simulink model "SEL_test"  (R2026a)
settings: Solver=ode8  StopTime=1  FixedStep=8e-9
PreLoadFcn:
  | setup_llrf
model workspace (MAT data in the model file):
  adc_sample_time = 8e-09
  alpha_ema = 0.00390625
  mag_Ki = 2000
  mag_Kp = 0.5
  max_dac_out = 1
  min_dac_out = 0
values from neighbouring files (symbols this model uses):
  f_IF = 10e6    (= 10000000)    [setup_llrf.m]
  f_sample = 125e6    (= 125000000)    [setup_llrf.m]
  lut_rSqrt = fi(lut_combined_float, 0, WL, FL, 'RoundingMethod', 'Nearest')    [LUT_gen.m]    (also in setup_llrf.m = LUT_gen)
  omega_0 = 2 * pi * f_IF    (= 62831853.0718)    [setup_llrf.m]
  omega_half = (f_0_rf / (2 * Q_L)) * 2 * pi    (= 8168.14089933)    [setup_llrf.m]
  params = extractHDLParams(filt)    [setup_llrf.m]
  t_sample = 1/f_sample    (= 8e-09)    [setup_llrf.m]
libraries: simulink x3, hdlsllib x2, dsphdlfiltering2 x2, dsphdlsigops2 x1
settings Model: DataTypeOverride=Off  FPTShortcutValueString='{{},{''BaselineRun'',1,1,1,''BaselineRun'','''',{},''M'',''D'',''''},{''BaselineRun_2'',1,1,1,''BaselineRun_2'','''',{},''M'',''D'',''''},{''EmbeddedRun'',1,1,1,''EmbeddedRun'','''',{},''M'','''',''''},{''EmbeddedRun_2'',1,1,1,''EmbeddedRun_2'','''',{},''M'','''',''''}}'  SnapshotInterval=1  Creator=Joshd  LastModifiedBy=Joshd
settings DataIOCC: InspectSignalLogs=on
settings OptimizationCC: ConditionallyExecuteInputs=off  InheritOutputTypeSmallerThanSingle=on
settings DebuggingCC: SignalRangeChecking=warning  ArtificialAlgebraicLoopMsg=error  SingleTaskRateTransMsg=error  UniqueDataStoreMsg=error  StrictBusMsg=ErrorOnBusTreatedAsVector
settings HardwareCC: ProdHWDeviceType=ASIC/FPGA->ASIC/FPGA  ProdEqTarget=off
settings ConfigComp: CovScope=ReferencedModels

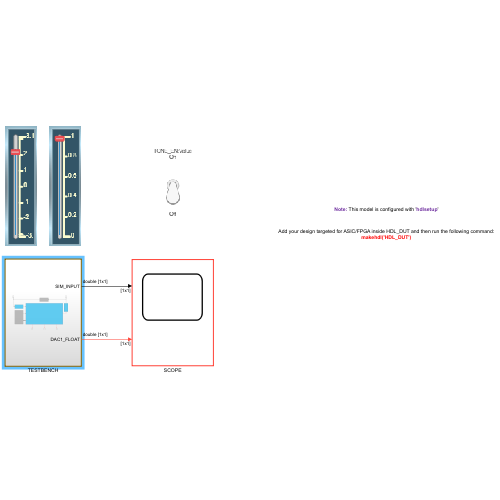
[thumbnail: Simulink's stored preview of the top-level diagram]
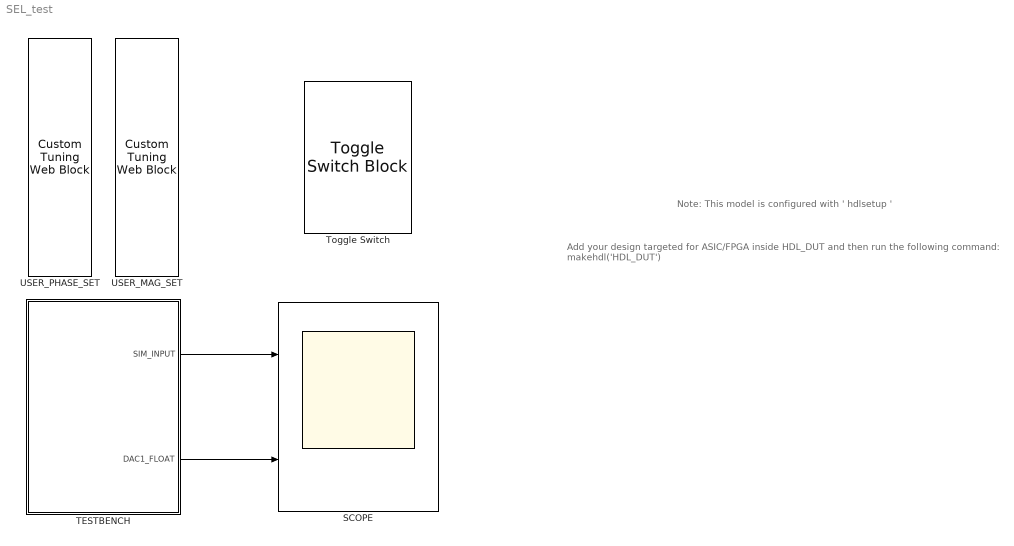
== system SEL_test ==
  note: Add your design targeted for ASIC/FPGA inside HDL_DUT and then run the following command:
      | makehdl('HDL_DUT')
  note: Note: This model is configured with ' hdlsetup '
  SCOPE : Scope  NumInputPorts=2
      settings: TimeSpan=1e-6  ActiveDisplayYMinimum=-2.1650361300192067  ActiveDisplayYMaximum=1.9862346787804239
  TESTBENCH : Subsystem
  Toggle Switch : ToggleSwitchBlock
  USER_MAG_SET : CustomTuningWebBlock  LabelPosition=Hide  ShowInitialText=on  Configuration="{\"components\":[{\"name\":\"LinearScaleComponent\",\"settings\":{\"bounds\":{\"max\":1,\"min\":0,\"tickInterval\":\"auto\"},\"internalTickHeightScaleFactor\":0.5,\"labelColor\":[255,255,200],\"labelFont\":{\"font\":\"Arial\",\"fontSize\":12},\"labelOffset\":0.05,\"labelTransparency\":1,\"needleImage\":{\"size\":[596,842],\"src\":\"data:image\\/svg+xml;base64,PD94bWwgdmVyc2lvbj0iMS4wIiBlbmNvZGluZz0idXRmLTgiPz4NCjwhLS0gR2VuZXJhdG9yOiBBZG9iZSBJbGx1c3RyYXRvciAyNS4wLjAsIFNWRyBFeHBvcnQgUGx1Zy1JbiAuIFNWRyBWZXJzaW9uOiA2LjAwIEJ1aWxkIDApICAtLT4NCjxzdmcgdmVyc2lvbj0iMS4xIg0KCSBpZD0ic3ZnOCIgeG1sbnM6Y2M9Imh0dHA6Ly9jcmVhdGl2ZWNvbW1vbnMub3JnL25zIyIgeG1sbnM6ZGM9Imh0dHA6Ly9wdXJsLm9yZy9kYy9lbGVtZW50cy8xLjEvIiB4bWxuczppbmtzY2FwZT0iaHR0cDovL3d3dy5pbmtzY2FwZS5vcmcvbmFtZXNw ...(+2420 chars)\",\"srcOrientation\":\"horizontal\"},\"needleOffset\":[0.0642123287671233,-0.8044596912521441],\"needleSize\":{\"height\":0.07668067226890757,\"width\":0.4337797619047619},\"position\":[0.03623949579831933,0.2829861111111111,0.6088789682539683,0.9196428571428571],\"referencePoint\":\"auto\",\"scaleColors\":[],\"scaleColorsSize\":0.2,\"scaleDirection\":\"BT\",\"showLabels\":1,\"showMinorTicks\":0,\"showSpanLine\":1,\"showTicks\":1,\"tickColor\":[252,252,197],\"tickTransparency\":1,\"valueBarColor\":[0,114,189],\"valueBarOffset\":-0.27,\"valueBarSize\":0.1,\"valueBarTransparency\":1}},{\"name\":\"BackgroundImageComponent\",\"settings\":{\"image\":{\"size\":[380,101],\"src\":\"data:image\\/svg+xml;base64,PHN2ZyB4bWxucz0iaHR0cDovL3d3dy53My5vcmcvMjAwMC9zdmciIHhtbG5zOnhsaW5rPSJodHRwOi8vd3d3LnczLm9yZy8xOTk5L3hsaW5rIiB2aWV3Qm94PSIwIDAgMzgwIDEwMSI+PGRlZnM+PHN0eWxlPi5jbHMtMXtmaWxsOiMwMDJiNDI7fS5jbHMtMntmaWxsOiM0MjcwODI7fS5jbHMtM3tmaWxsOnVybCgjcmFkaWFsLWdyYWRpZW50KTt9LmNscy00e2ZpbGw6I2M4YzhjODtzdHJva2U6IzAwMDt9PC9zdHlsZT48cmFkaWFsR3JhZGllbnQgaWQ9InJhZGlhbC1ncmFkaWVudCIgY3g9IjE5MCIgY3k9IjUwLjUiIHI9IjI2OS4yMSIgZ3JhZGllbnRVbml0cz0idXNlclNwYWNlT25Vc2UiPjxzdG9wIG9mZnNldD0iMC4wMSIgc3RvcC1jb2xvcj0iIzNlNGY1OCIvPjxzdG9wIG9mZnNldD0iMC4wNiIgc3RvcC1jb2xvcj0iIzQ0NTc2MSIvPjxzdG9wIG9mZnNldD0iMC4xNSIgc3RvcC1jb2xvcj0iIzU1NmE3NiIvPjxzdG9wIG9mZnNldD0iMC4yNSIgc3RvcC1jb2xvcj0iIzZkODg5NSIvPjxzdG9wIG9mZnNldD0iMC4zOCIgc3RvcC1jb2xvcj0iIzhmYjJjMyIvPjxzdG9wIG9mZnNldD0iMC41MiIgc3RvcC1jb2xvcj0iI2I2ZTRmYSIvPjxzdG9wIG9mZnNldD0iMSIgc3RvcC1jb2xvcj0iIzE1NDY1NyIvPjwvcmFkaWFsR3JhZGllbnQ+PC9kZWZzPjxnIGlkPSJmcmFtZSI+PGcgaWQ9IkxheWVyXzIiIGRhdGEtbmFtZT0iTGF5ZXIgMiI+PGcgaWQ9IkxheWVyXzEtMiIgZGF0YS1uYW1lPSJMYXllciAxLTIiPjxyZWN0IGlkPSJyZWN0MTAzNiIgY2xhc3M9ImNscy0xIiB4PSIxMSIgeT0iMTEiIHdpZHRoPSIzNTgiIGhlaWdodD0iNzkiLz48cGF0aCBpZD0icGF0aDEwMzgiIGNsYXNzPSJjbHMtMiIgZD0iTTgsOFY5M0gzNzJWOFpNMzY5LDkwSDExVjExSDM2OVoiLz48cGF0aCBpZD0icGF0aDEwNDAiIGNsYXNzPSJjbHMtMyIgZD0iTTAsMFYxMDFIMzgwVjBaTTM3Miw5M0g4VjhIMzcyWiIvPjwvZz48L2c+PC9nPjxnIGlkPSJ0cmFjayI+PHBhdGggaWQ9InJlY3QxNjExIiBjbGFzcz0iY2xzLTQiIGQ9Ik0zMy4zNywyNi41OUgzNDYuNjNjNCwwLDcuMjUsMi42LDcuMjUsNS44MWgwYzAsMy4yMS0zLjI1LDUuODItNy4yNSw1LjgySDMzLjM3Yy00LDAtNy4yNS0yLjYxLTcuMjUtNS44MmgwQzI2LjEyLDI5LjE5LDI5LjM3LDI2LjU5LDMzLjM3LDI2LjU5WiIvPjwvZz48L3N2Zz4=\",\"srcOrientation\":\"horizontal\"},\"position\":[0,0,1,1],\"scaleMode\":\"0\"}},{\"name\":\"ForegroundImageComponent\",\"settings\":{\"image\":{\"size\":[0,0],\"src\":\"default\",\"srcOrientation\":[]},\"isForeground\":1,\"position\":[0,0,1,1],\"scaleMode\":\"0\"}}],\"derived\":{\"blockParameters\":{\"ForegroundColor\":[0.9882352941176471,0.9882352941176471,0.7725490196078432],\"Limits\":{\"Max\":1,\"Min\":0,\"Ticks\":\"auto\"},\"ScaleColors\":[],\"ScaleDirection\":\"Clockwise\",\"ScaleMax\":1,\"ScaleMin\":0,\"TickInterval\":\"auto\",\"fixedAspectRatio\":\"on\"}},\"settings\":{\"BindingType\":\"param\",\"aspectRatio\":3.7777777777777777,\"backgroundColor\":[0,0,0,\"1\"],\"backgroundOffset\":0,\"backgroundOpacity\":1,\"fixedAspectRatio\":\"on\",\"foregroundColor\":[252,252,196],\"orientation\":\"vertical\",\"showBackgroundColor\":false,\"value\":0,\"version\":\"R2023a\"},\"type\":\"LinearGauge\"}"
  USER_PHASE_SET : CustomTuningWebBlock  LabelPosition=Hide  ShowInitialText=on  Configuration="{\"components\":[{\"name\":\"LinearScaleComponent\",\"settings\":{\"bounds\":{\"max\":3.14159,\"min\":-3.14159,\"tickInterval\":\"auto\"},\"internalTickHeightScaleFactor\":0.5,\"labelColor\":[255,255,200],\"labelFont\":{\"font\":\"Arial\",\"fontSize\":12},\"labelOffset\":0.05,\"labelTransparency\":1,\"needleImage\":{\"size\":[596,842],\"src\":\"data:image\\/svg+xml;base64,PD94bWwgdmVyc2lvbj0iMS4wIiBlbmNvZGluZz0idXRmLTgiPz4NCjwhLS0gR2VuZXJhdG9yOiBBZG9iZSBJbGx1c3RyYXRvciAyNS4wLjAsIFNWRyBFeHBvcnQgUGx1Zy1JbiAuIFNWRyBWZXJzaW9uOiA2LjAwIEJ1aWxkIDApICAtLT4NCjxzdmcgdmVyc2lvbj0iMS4xIg0KCSBpZD0ic3ZnOCIgeG1sbnM6Y2M9Imh0dHA6Ly9jcmVhdGl2ZWNvbW1vbnMub3JnL25zIyIgeG1sbnM6ZGM9Imh0dHA6Ly9wdXJsLm9yZy9kYy9lbGVtZW50cy8xLjEvIiB4bWxuczppbmtzY2FwZT0iaHR0cDovL3d3dy5pbmtzY2FwZS5vcmcvbmFtZXNw ...(+2420 chars)\",\"srcOrientation\":\"horizontal\"},\"needleOffset\":[0.0642123287671233,-0.8044596912521441],\"needleSize\":{\"height\":0.07668067226890757,\"width\":0.4337797619047619},\"position\":[0.03623949579831933,0.2829861111111111,0.6088789682539683,0.9196428571428571],\"referencePoint\":\"auto\",\"scaleColors\":[],\"scaleColorsSize\":0.2,\"scaleDirection\":\"BT\",\"showLabels\":1,\"showMinorTicks\":0,\"showSpanLine\":1,\"showTicks\":1,\"tickColor\":[252,252,197],\"tickTransparency\":1,\"valueBarColor\":[0,114,189],\"valueBarOffset\":-0.27,\"valueBarSize\":0.1,\"valueBarTransparency\":1}},{\"name\":\"BackgroundImageComponent\",\"settings\":{\"image\":{\"size\":[380,101],\"src\":\"data:image\\/svg+xml;base64,PHN2ZyB4bWxucz0iaHR0cDovL3d3dy53My5vcmcvMjAwMC9zdmciIHhtbG5zOnhsaW5rPSJodHRwOi8vd3d3LnczLm9yZy8xOTk5L3hsaW5rIiB2aWV3Qm94PSIwIDAgMzgwIDEwMSI+PGRlZnM+PHN0eWxlPi5jbHMtMXtmaWxsOiMwMDJiNDI7fS5jbHMtMntmaWxsOiM0MjcwODI7fS5jbHMtM3tmaWxsOnVybCgjcmFkaWFsLWdyYWRpZW50KTt9LmNscy00e2ZpbGw6I2M4YzhjODtzdHJva2U6IzAwMDt9PC9zdHlsZT48cmFkaWFsR3JhZGllbnQgaWQ9InJhZGlhbC1ncmFkaWVudCIgY3g9IjE5MCIgY3k9IjUwLjUiIHI9IjI2OS4yMSIgZ3JhZGllbnRVbml0cz0idXNlclNwYWNlT25Vc2UiPjxzdG9wIG9mZnNldD0iMC4wMSIgc3RvcC1jb2xvcj0iIzNlNGY1OCIvPjxzdG9wIG9mZnNldD0iMC4wNiIgc3RvcC1jb2xvcj0iIzQ0NTc2MSIvPjxzdG9wIG9mZnNldD0iMC4xNSIgc3RvcC1jb2xvcj0iIzU1NmE3NiIvPjxzdG9wIG9mZnNldD0iMC4yNSIgc3RvcC1jb2xvcj0iIzZkODg5NSIvPjxzdG9wIG9mZnNldD0iMC4zOCIgc3RvcC1jb2xvcj0iIzhmYjJjMyIvPjxzdG9wIG9mZnNldD0iMC41MiIgc3RvcC1jb2xvcj0iI2I2ZTRmYSIvPjxzdG9wIG9mZnNldD0iMSIgc3RvcC1jb2xvcj0iIzE1NDY1NyIvPjwvcmFkaWFsR3JhZGllbnQ+PC9kZWZzPjxnIGlkPSJmcmFtZSI+PGcgaWQ9IkxheWVyXzIiIGRhdGEtbmFtZT0iTGF5ZXIgMiI+PGcgaWQ9IkxheWVyXzEtMiIgZGF0YS1uYW1lPSJMYXllciAxLTIiPjxyZWN0IGlkPSJyZWN0MTAzNiIgY2xhc3M9ImNscy0xIiB4PSIxMSIgeT0iMTEiIHdpZHRoPSIzNTgiIGhlaWdodD0iNzkiLz48cGF0aCBpZD0icGF0aDEwMzgiIGNsYXNzPSJjbHMtMiIgZD0iTTgsOFY5M0gzNzJWOFpNMzY5LDkwSDExVjExSDM2OVoiLz48cGF0aCBpZD0icGF0aDEwNDAiIGNsYXNzPSJjbHMtMyIgZD0iTTAsMFYxMDFIMzgwVjBaTTM3Miw5M0g4VjhIMzcyWiIvPjwvZz48L2c+PC9nPjxnIGlkPSJ0cmFjayI+PHBhdGggaWQ9InJlY3QxNjExIiBjbGFzcz0iY2xzLTQiIGQ9Ik0zMy4zNywyNi41OUgzNDYuNjNjNCwwLDcuMjUsMi42LDcuMjUsNS44MWgwYzAsMy4yMS0zLjI1LDUuODItNy4yNSw1LjgySDMzLjM3Yy00LDAtNy4yNS0yLjYxLTcuMjUtNS44MmgwQzI2LjEyLDI5LjE5LDI5LjM3LDI2LjU5LDMzLjM3LDI2LjU5WiIvPjwvZz48L3N2Zz4=\",\"srcOrientation\":\"horizontal\"},\"position\":[0,0,1,1],\"scaleMode\":\"0\"}},{\"name\":\"ForegroundImageComponent\",\"settings\":{\"image\":{\"size\":[0,0],\"src\":\"default\",\"srcOrientation\":[]},\"isForeground\":1,\"position\":[0,0,1,1],\"scaleMode\":\"0\"}}],\"derived\":{\"blockParameters\":{\"ForegroundColor\":[0.9882352941176471,0.9882352941176471,0.7725490196078432],\"Limits\":{\"Max\":3.14159,\"Min\":-3.14159,\"Ticks\":\"auto\"},\"ScaleColors\":[],\"ScaleDirection\":\"Clockwise\",\"ScaleMax\":3.14159,\"ScaleMin\":-3.14159,\"TickInterval\":\"auto\",\"fixedAspectRatio\":\"on\"}},\"settings\":{\"BindingType\":\"param\",\"aspectRatio\":3.7777777777777777,\"backgroundColor\":[0,0,0,\"1\"],\"backgroundOffset\":0,\"backgroundOpacity\":1,\"fixedAspectRatio\":\"on\",\"foregroundColor\":[252,252,196],\"orientation\":\"vertical\",\"showBackgroundColor\":false,\"value\":0,\"version\":\"R2023a\"},\"type\":\"LinearGauge\"}"
  wires:
  TESTBENCH/1(SIM_INPUT) -> SCOPE/1
  TESTBENCH/2(DAC1_FLOAT) -> SCOPE/2

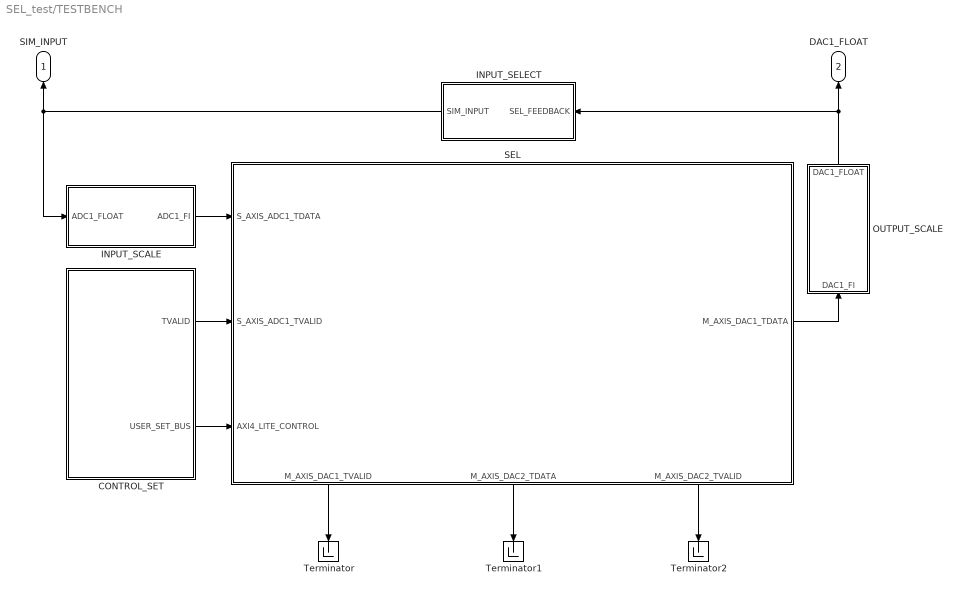
== system SEL_test/TESTBENCH ==
  CONTROL_SET : Subsystem
  INPUT_SCALE : Subsystem
  INPUT_SELECT : Subsystem
  OUTPUT_SCALE : Subsystem
  SEL : Subsystem  TreatAsAtomicUnit=on
      settings: PortSchema="{\"entries\":[{\"content\":{\"sides\":[{\"content\":{\"connectorIds\":[\"In1\",\"In2\",\"In3\"]},\"type\":\"ConnectorPlacement.EquallySpacedRectSide\",\"uuid\":\"33e7de77-9901-449c-9630-f09cdbbbff97\"},{\"content\":{\"connectorIds\":[\"Out1\"],\"side\":\"RIGHT\"},\"type\":\"ConnectorPlacement.EquallySpacedRectSide\",\"uuid\":\"be4966c7-0cb0-4620-90c7-b485869ca97c\"},{\"content\":{\"side\":\"TOP\"},\"type\":\"ConnectorPlacement.EquallySpacedRectSide\",\"uuid\":\"879d56ef-4ddc-415a-a20c-e3a6815a11d0\"},{\"content\":{\"connectorIds\":[\"Out2\",\"Out3\",\"Out4\"],\"side\":\"BOTTOM\"},\"type\":\"ConnectorPlacement.EquallySpacedRectSide\",\"uuid\":\"4f2a598c-be1d-44e7-8b71-9487e2bf94fb\"}]},\"type\":\"ConnectorPlacement.EquallySpacedConnector\",\"uuid\":\"cba36172-b30a-4b6d-840d-8fe0281760af\"}],\"packageUris\":[\"http://schema.mathworks.com/mf0/Connector/R2020b\"],\"version\":\"1.0\"}"
  Terminator : Terminator
  Terminator1 : Terminator
  Terminator2 : Terminator
  SIM_INPUT : Outport
  DAC1_FLOAT : Outport  Port=2
  wires:
  INPUT_SCALE/1(ADC1_FI) -> SEL/1(S_AXIS_ADC1_TDATA)
  SEL/1(M_AXIS_DAC1_TDATA) -> OUTPUT_SCALE/1(DAC1_FI)
  CONTROL_SET/1(TVALID) -> SEL/2(S_AXIS_ADC1_TVALID)
  CONTROL_SET/2(USER_SET_BUS) -> SEL/3(AXI4_LITE_CONTROL)
  INPUT_SELECT/1(SIM_INPUT) -> INPUT_SCALE/1(ADC1_FLOAT), SIM_INPUT/1
  OUTPUT_SCALE/1(DAC1_FLOAT) -> INPUT_SELECT/1(SEL_FEEDBACK), DAC1_FLOAT/1
  SEL/4(M_AXIS_DAC2_TVALID) -> Terminator2/1
  SEL/3(M_AXIS_DAC2_TDATA) -> Terminator1/1
  SEL/2(M_AXIS_DAC1_TVALID) -> Terminator/1

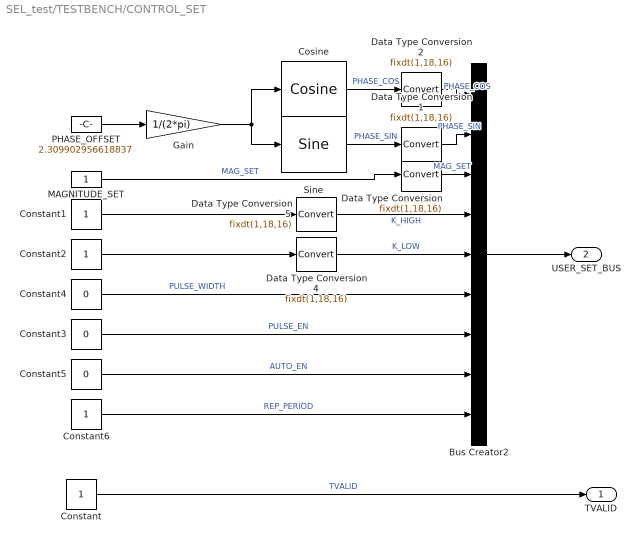
== system SEL_test/TESTBENCH/CONTROL_SET ==
  Bus Creator2 : BusCreator  Inputs=9
  Constant : Constant  OutDataTypeStr=boolean
  Constant1 : Constant  SampleTime=t_sample
  Constant2 : Constant  SampleTime=t_sample
  Constant3 : Constant  Value=0  OutDataTypeStr=boolean  SampleTime=t_sample
  Constant4 : Constant  Value=0  OutDataTypeStr=uint32
  Constant5 : Constant  Value=0  OutDataTypeStr=boolean
  Constant6 : Constant  OutDataTypeStr=uint32
  Cosine : simulink/Lookup Tables/Cosine  Formula=cos(2*pi*u)  NumDataPoints=(2^5)+1  OutputWordLength=18  InternalRulePriority=Speed
  Data Type Conversion{,1..2,4..5} (5 alike) : DataTypeConversion  OutDataTypeStr=fixdt(1,18,16)  RndMeth=Nearest
  Gain : Gain  Gain=1/(2*pi)
  MAGNITUDE_SET : Constant  SampleTime=t_sample
  PHASE_OFFSET : Constant  Value=2.309902956618837  SampleTime=t_sample
  Sine : simulink/Lookup Tables/Sine  Formula=sin(2*pi*u)  NumDataPoints=(2^5)+1  OutputWordLength=18  InternalRulePriority=Speed
  TVALID : Outport
  USER_SET_BUS : Outport  Port=2
  wires:
  Constant/1 -> TVALID/1  "TVALID"
  PHASE_OFFSET/1 -> Gain/1
  Gain/1 -> Cosine/1, Sine/1
  Sine/1 -> Data Type Conversion1/1  "PHASE_SIN"
  MAGNITUDE_SET/1 -> Data Type Conversion/1  "MAG_SET"
  Cosine/1 -> Data Type Conversion2/1  "PHASE_COS"
  Data Type Conversion2/1 -> Bus Creator2/1  "PHASE_COS"
  Data Type Conversion1/1 -> Bus Creator2/2  "PHASE_SIN"
  Data Type Conversion/1 -> Bus Creator2/3  "MAG_SET"
  Bus Creator2/1 -> USER_SET_BUS/1
  Constant3/1 -> Bus Creator2/7  "PULSE_EN"
  Constant2/1 -> Data Type Conversion4/1
  Constant1/1 -> Data Type Conversion5/1
  Data Type Conversion5/1 -> Bus Creator2/4  "K_HIGH"
  Data Type Conversion4/1 -> Bus Creator2/5  "K_LOW"
  Constant4/1 -> Bus Creator2/6  "PULSE_WIDTH"
  Constant6/1 -> Bus Creator2/9  "REP_PERIOD"
  Constant5/1 -> Bus Creator2/8  "AUTO_EN"

== system SEL_test/TESTBENCH/INPUT_SCALE ==
  ADC1_FLOAT : Inport
  Gain1 : Gain  Gain=8192 * 4
  SEL_boundary_DTC : DataTypeConversion  OutDataTypeStr=fixdt(1,16,0)  RndMeth=Nearest
  ADC1_FI : Outport
  wires:
  Gain1/1 -> SEL_boundary_DTC/1
  ADC1_FLOAT/1 -> Gain1/1
  SEL_boundary_DTC/1 -> ADC1_FI/1  "TDATA"

== system SEL_test/TESTBENCH/INPUT_SELECT ==
  SEL_FEEDBACK : Inport
  CAVITY_SIM : TransferFcn  Numerator=[2*omega_half, 0]  Denominator=[1, 2 * omega_half, omega_0^2]
  Sum : Sum  Inputs=|++
  Switch : Switch  Criteria=u2 ~= 0  SaturateOnIntegerOverflow=off  InputSameDT=off
  THERMAL_NOISE : simulink/Sources/Band-Limited White Noise  Cov=3e-12  Ts=t_sample  seed=[23341]
  TONE : Sin  Frequency=10*2*pi*1e6  SampleTime=0
  TONE_EN : Constant  Value=0
  SIM_INPUT : Outport
  wires:
  CAVITY_SIM/1 -> Switch/3
  TONE_EN/1 -> Switch/2
  THERMAL_NOISE/1 -> Sum/1
  TONE/1 -> Switch/1
  Sum/1 -> CAVITY_SIM/1
  Switch/1 -> SIM_INPUT/1
  SEL_FEEDBACK/1 -> Sum/2

== system SEL_test/TESTBENCH/OUTPUT_SCALE ==
  DAC1_FI : Inport
  Bus Selector : BusSelector  OutputSignals=TDATA
  Gain2 : Gain  Gain=1/32768  OutDataTypeStr=double
  DAC1_FLOAT : Outport
  wires:
  Bus Selector/1 -> Gain2/1  "<TDATA>"
  Gain2/1 -> DAC1_FLOAT/1
  DAC1_FI/1 -> Bus Selector/1

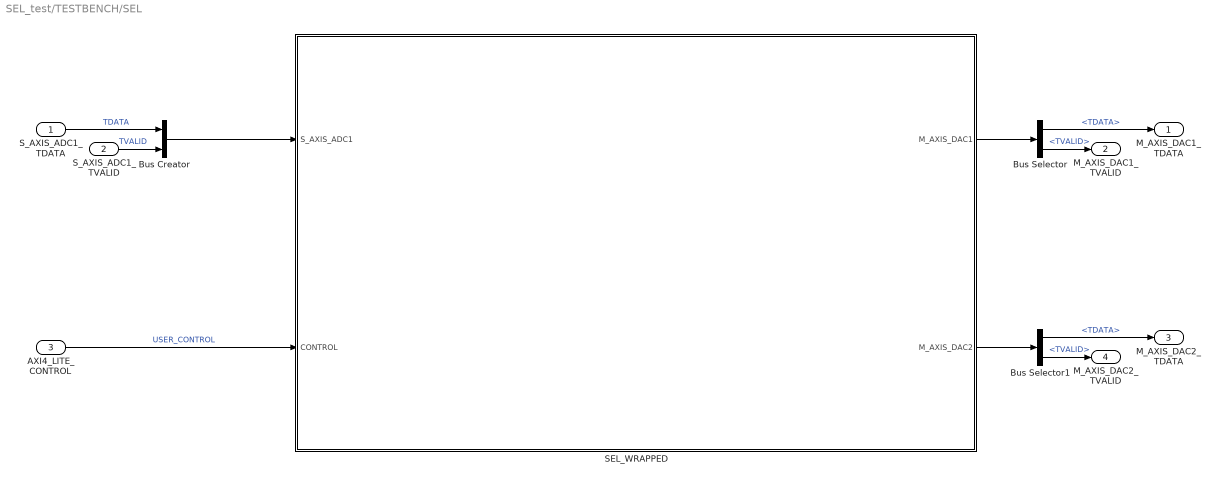
== system SEL_test/TESTBENCH/SEL ==
  S_AXIS_ADC1_TDATA : Inport  OutMin=-32768  OutMax=32767  SampleTime=t_sample  LockScale=on
  S_AXIS_ADC1_TVALID : Inport  Port=2  SampleTime=t_sample
  AXI4_LITE_CONTROL : Inport  Port=3  SampleTime=t_sample
  Bus Creator : BusCreator  Inputs=2
  Bus Selector : BusSelector  OutputSignals=TDATA,TVALID
  Bus Selector1 : BusSelector  OutputSignals=TDATA,TVALID
  SEL_WRAPPED : Subsystem
  M_AXIS_DAC1_TDATA : Outport  OutMin=-32768  OutMax=32767  VectorParamsAs1DForOutWhenUnconnected=off  LockScale=on
  M_AXIS_DAC1_TVALID : Outport  Port=2  VectorParamsAs1DForOutWhenUnconnected=off
  M_AXIS_DAC2_TDATA : Outport  Port=3  VectorParamsAs1DForOutWhenUnconnected=off
  M_AXIS_DAC2_TVALID : Outport  Port=4  VectorParamsAs1DForOutWhenUnconnected=off
  wires:
  AXI4_LITE_CONTROL/1 -> SEL_WRAPPED/2(CONTROL)  "USER_CONTROL"
  SEL_WRAPPED/1(M_AXIS_DAC1) -> Bus Selector/1
  S_AXIS_ADC1_TDATA/1 -> Bus Creator/1  "TDATA"
  S_AXIS_ADC1_TVALID/1 -> Bus Creator/2  "TVALID"
  Bus Creator/1 -> SEL_WRAPPED/1(S_AXIS_ADC1)
  Bus Selector/1 -> M_AXIS_DAC1_TDATA/1  "<TDATA>"
  Bus Selector/2 -> M_AXIS_DAC1_TVALID/1  "<TVALID>"
  SEL_WRAPPED/2(M_AXIS_DAC2) -> Bus Selector1/1
  Bus Selector1/1 -> M_AXIS_DAC2_TDATA/1  "<TDATA>"
  Bus Selector1/2 -> M_AXIS_DAC2_TVALID/1  "<TVALID>"

== system SEL_test/TESTBENCH/SEL/SEL_WRAPPED ==
  note: DAC1
  note: DAC2
  note: ADC1
  note: CONTROL
  S_AXIS_ADC1 : Inport  SampleTime=t_sample  LockScale=on
  CONTROL : Inport  Port=2  SampleTime=t_sample
  DSP_LOGIC : Subsystem
      settings: PortSchema="{\"entries\":[{\"content\":{\"sides\":[{\"content\":{\"connectorIds\":[\"In1\"]},\"type\":\"ConnectorPlacement.EquallySpacedRectSide\",\"uuid\":\"317db4af-ec8e-456f-912c-3d65e229fa2f\"},{\"content\":{\"connectorIds\":[\"Out1\"],\"side\":\"RIGHT\"},\"type\":\"ConnectorPlacement.EquallySpacedRectSide\",\"uuid\":\"b87d0049-b55a-42e6-8fe3-835706ccf696\"},{\"content\":{\"side\":\"TOP\"},\"type\":\"ConnectorPlacement.EquallySpacedRectSide\",\"uuid\":\"9ac7dae0-4538-4c40-8de7-0e66e4db1f0a\"},{\"content\":{\"connectorIds\":[\"In2\"],\"side\":\"BOTTOM\"},\"type\":\"ConnectorPlacement.EquallySpacedRectSide\",\"uuid\":\"fe5d993e-d69e-450a-a884-182e0cabd30d\"}]},\"type\":\"ConnectorPlacement.EquallySpacedConnector\",\"uuid\":\"e3931264-6d81-40f1-85ac-623eb179009f\"}],\"packageUris\":[\"http://schema.mathworks.com/mf0/Connector/R2020b\"],\"version\":\"1.0\"}"
  M_AXIS_DAC1 : Outport  SampleTime=t_sample  VectorParamsAs1DForOutWhenUnconnected=off  LockScale=on
  M_AXIS_DAC2 : Outport  Port=2  VectorParamsAs1DForOutWhenUnconnected=off
  wires:
  CONTROL/1 -> DSP_LOGIC/2(AXI_LITE_CONTROL)
  DSP_LOGIC/1(DAC1_OUT) -> M_AXIS_DAC1/1
  S_AXIS_ADC1/1 -> M_AXIS_DAC2/1, DSP_LOGIC/1(ADC1_IN)

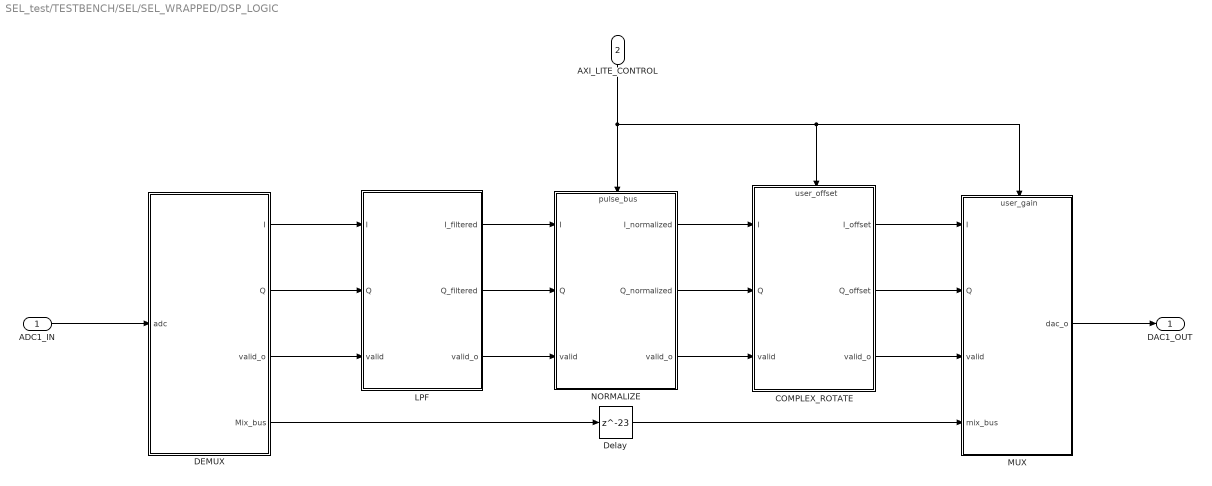
== system SEL_test/TESTBENCH/SEL/SEL_WRAPPED/DSP_LOGIC ==
  ADC1_IN : Inport
  AXI_LITE_CONTROL : Inport  Port=2
  COMPLEX_ROTATE : Subsystem
      settings: PortSchema="{\"entries\":[{\"content\":{\"sides\":[{\"content\":{\"connectorIds\":[\"In1\",\"In2\",\"In3\"]},\"type\":\"ConnectorPlacement.EquallySpacedRectSide\",\"uuid\":\"d51fc2b3-d39d-452f-8834-c00ba2a7647d\"},{\"content\":{\"connectorIds\":[\"Out1\",\"Out2\",\"Out3\"],\"side\":\"RIGHT\"},\"type\":\"ConnectorPlacement.EquallySpacedRectSide\",\"uuid\":\"1966010c-3348-463c-9cb9-88942c557d5a\"},{\"content\":{\"connectorIds\":[\"In4\"],\"side\":\"TOP\"},\"type\":\"ConnectorPlacement.EquallySpacedRectSide\",\"uuid\":\"4d882d03-7803-4123-88b9-cc4c11464e72\"}]},\"type\":\"ConnectorPlacement.EquallySpacedConnector\",\"uuid\":\"18216865-41d8-4679-a806-f2149c408dc2\"}],\"packageUris\":[\"http://schema.mathworks.com/mf0/Connector/R2020b\"],\"version\":\"1.0\"}"
  DEMUX : Subsystem  TreatAsAtomicUnit=on
  Delay : Delay  DelayLength=23  InitialCondition=0
  LPF : Subsystem  TreatAsAtomicUnit=on
  MUX : Subsystem
      settings: PortSchema="{\"entries\":[{\"content\":{\"sides\":[{\"content\":{\"connectorIds\":[\"In1\",\"In2\",\"In3\",\"In4\"]},\"type\":\"ConnectorPlacement.EquallySpacedRectSide\",\"uuid\":\"d65dacbd-4698-4e58-a804-f5cf1967e0ff\"},{\"content\":{\"connectorIds\":[\"Out1\"],\"side\":\"RIGHT\"},\"type\":\"ConnectorPlacement.EquallySpacedRectSide\",\"uuid\":\"24eef561-fd60-4956-8955-03b42f279571\"},{\"content\":{\"connectorIds\":[\"In5\"],\"side\":\"TOP\"},\"type\":\"ConnectorPlacement.EquallySpacedRectSide\",\"uuid\":\"d3a23786-0d53-4abc-a8bf-9ada5994f835\"}]},\"type\":\"ConnectorPlacement.EquallySpacedConnector\",\"uuid\":\"1b44fd2c-4087-4f3f-a0ee-f41bc0205dd0\"}],\"packageUris\":[\"http://schema.mathworks.com/mf0/Connector/R2020b\"],\"version\":\"1.0\"}"
  NORMALIZE : Subsystem
      settings: PortSchema="{\"entries\":[{\"content\":{\"sides\":[{\"content\":{\"connectorIds\":[\"In1\",\"In2\",\"In3\"]},\"type\":\"ConnectorPlacement.EquallySpacedRectSide\",\"uuid\":\"eba04924-33b5-497a-994b-57365ff34f04\"},{\"content\":{\"connectorIds\":[\"Out1\",\"Out2\",\"Out3\"],\"side\":\"RIGHT\"},\"type\":\"ConnectorPlacement.EquallySpacedRectSide\",\"uuid\":\"221a6795-cbc8-48b7-aad4-8d3ce17f65fa\"},{\"content\":{\"connectorIds\":[\"In4\"],\"side\":\"TOP\"},\"type\":\"ConnectorPlacement.EquallySpacedRectSide\",\"uuid\":\"357064fa-6532-4ccc-9363-4fd2750b7b1b\"}]},\"type\":\"ConnectorPlacement.EquallySpacedConnector\",\"uuid\":\"cc651dc9-aa3d-4457-a645-2b2a77ecb91e\"}],\"packageUris\":[\"http://schema.mathworks.com/mf0/Connector/R2020b\"],\"version\":\"1.0\"}"
  DAC1_OUT : Outport
  wires:
  MUX/1(dac_o) -> DAC1_OUT/1
  DEMUX/2(Q) -> LPF/2(Q)
  DEMUX/1(I) -> LPF/1(I)
  DEMUX/3(valid_o) -> LPF/3(valid)
  ADC1_IN/1 -> DEMUX/1(adc)
  DEMUX/4(Mix_bus) -> Delay/1
  LPF/3(valid_o) -> NORMALIZE/3(valid)
  NORMALIZE/3(valid_o) -> COMPLEX_ROTATE/3(valid)
  NORMALIZE/2(Q_normalized) -> COMPLEX_ROTATE/2(Q)
  COMPLEX_ROTATE/3(valid_o) -> MUX/3(valid)
  COMPLEX_ROTATE/2(Q_offset) -> MUX/2(Q)
  NORMALIZE/1(I_normalized) -> COMPLEX_ROTATE/1(I)
  COMPLEX_ROTATE/1(I_offset) -> MUX/1(I)
  Delay/1 -> MUX/4(mix_bus)
  LPF/1(I_filtered) -> NORMALIZE/1(I)
  LPF/2(Q_filtered) -> NORMALIZE/2(Q)
  AXI_LITE_CONTROL/1 -> MUX/5(user_gain), COMPLEX_ROTATE/4(user_offset), NORMALIZE/4(pulse_bus)

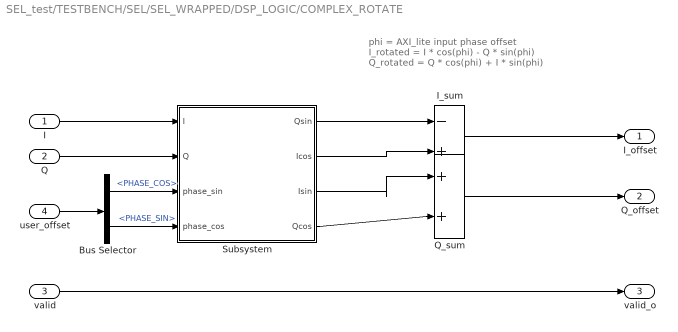
== system SEL_test/TESTBENCH/SEL/SEL_WRAPPED/DSP_LOGIC/COMPLEX_ROTATE ==
  note: phi = AXI_lite input phase offset
      | I_rotated = I * cos(phi) - Q * sin(phi)
      | Q_rotated = Q * cos(phi) + I * sin(phi)
  I : Inport
  Q : Inport  Port=2
  valid : Inport  Port=3
  user_offset : Inport  Port=4
  Bus Selector : BusSelector  OutputSignals=PHASE_COS,PHASE_SIN
  I_sum : Sum  Inputs=-+  RndMeth=Nearest  SaturateOnIntegerOverflow=on
  Q_sum : Sum  Inputs=|++  RndMeth=Nearest  SaturateOnIntegerOverflow=on
  Subsystem : Subsystem
  I_offset : Outport
  Q_offset : Outport  Port=2  VectorParamsAs1DForOutWhenUnconnected=off
  valid_o : Outport  Port=3  VectorParamsAs1DForOutWhenUnconnected=off
  wires:
  I_sum/1 -> I_offset/1
  Q_sum/1 -> Q_offset/1
  valid/1 -> valid_o/1
  I/1 -> Subsystem/1(I)
  Q/1 -> Subsystem/2(Q)
  Subsystem/1(Qsin) -> I_sum/1
  Subsystem/2(Icos) -> I_sum/2
  Subsystem/3(Isin) -> Q_sum/1
  Subsystem/4(Qcos) -> Q_sum/2
  user_offset/1 -> Bus Selector/1
  Bus Selector/1 -> Subsystem/3(phase_sin)  "<PHASE_COS>"
  Bus Selector/2 -> Subsystem/4(phase_cos)  "<PHASE_SIN>"

== system SEL_test/TESTBENCH/SEL/SEL_WRAPPED/DSP_LOGIC/DEMUX ==
  adc : Inport
  MIX : Subsystem
  NCO : Subsystem
  I : Outport
  Q : Outport  Port=2
  valid_o : Outport  Port=3
  Mix_bus : Outport  Port=4  VectorParamsAs1DForOutWhenUnconnected=off
  wires:
  adc/1 -> MIX/1(adc_in)
  NCO/1(mix_bus_out) -> MIX/2(mix_bus_in)
  MIX/1(Q_mix1) -> Q/1
  MIX/2(I_mixed) -> I/1
  MIX/3(mix_bus_out) -> Mix_bus/1
  NCO/2(valid_out) -> MIX/3(valid_in)
  MIX/4(valid_out) -> valid_o/1

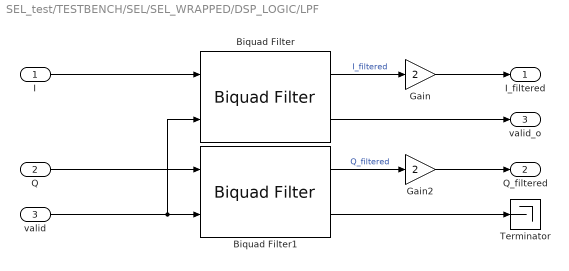
== system SEL_test/TESTBENCH/SEL/SEL_WRAPPED/DSP_LOGIC/LPF ==
  I : Inport
  Q : Inport  Port=2
  valid : Inport  Port=3
  Biquad Filter : dsphdlfiltering2/Biquad Filter  Structure=Pipelined feedback form  Numerator=params.Num  Denominator=params.Den  ScaleValues=params.g  SimulateUsing=Code generation  roundingMode=Nearest  overflowMode=on  NumeratorDataTypeStr=fixdt(1,25,23)  DenominatorDataTypeStr=fixdt(1,25,23)  ScaleValuesDataTypeStr=fixdt(1,25,23)  CoefficientsDataTypeStr=Inherit: Same word length as input  AccumulatorDataTypeStr=fixdt(1,48,38)  OutputDataTypeStr=fixdt(1,25,23)
  Biquad Filter1 : dsphdlfiltering2/Biquad Filter  Structure=Pipelined feedback form  Numerator=params.Num  Denominator=params.Den  ScaleValues=params.g  SimulateUsing=Code generation  roundingMode=Nearest  overflowMode=on  NumeratorDataTypeStr=fixdt(1,25,23)  DenominatorDataTypeStr=fixdt(1,25,23)  ScaleValuesDataTypeStr=fixdt(1,25,23)  CoefficientsDataTypeStr=Inherit: Same word length as input  AccumulatorDataTypeStr=fixdt(1,48,38)  OutputDataTypeStr=fixdt(1,25,23)
  Gain : Gain  Gain=2  RndMeth=Nearest  SaturateOnIntegerOverflow=on  OutDataTypeStr=Inherit: Same as input
  Gain2 : Gain  Gain=2  RndMeth=Nearest  SaturateOnIntegerOverflow=on  OutDataTypeStr=Inherit: Same as input
  Terminator : Terminator
  I_filtered : Outport  OutMin=-1  OutMax=.999
  Q_filtered : Outport  Port=2  OutMin=-1  OutMax=.999
  valid_o : Outport  Port=3  VectorParamsAs1DForOutWhenUnconnected=off
  wires:
  Biquad Filter/1 -> Gain/1  "I_filtered"
  Biquad Filter/2 -> valid_o/1
  Biquad Filter1/2 -> Terminator/1
  valid/1 -> Biquad Filter1/2, Biquad Filter/2
  I/1 -> Biquad Filter/1
  Biquad Filter1/1 -> Gain2/1  "Q_filtered"
  Q/1 -> Biquad Filter1/1
  Gain/1 -> I_filtered/1
  Gain2/1 -> Q_filtered/1

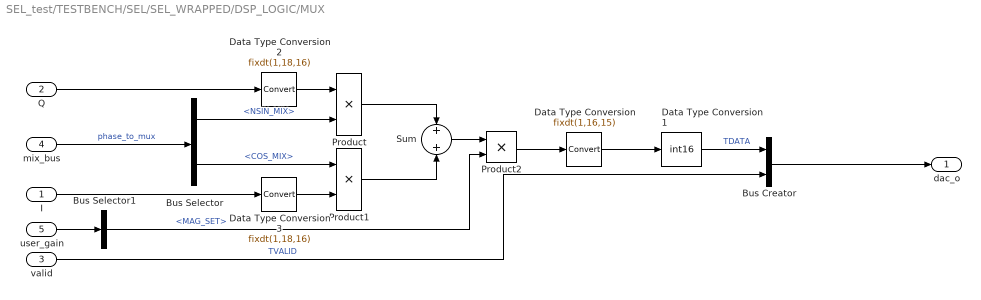
== system SEL_test/TESTBENCH/SEL/SEL_WRAPPED/DSP_LOGIC/MUX ==
  I : Inport  SampleTime=t_sample
  Q : Inport  Port=2  SampleTime=t_sample
  valid : Inport  Port=3
  mix_bus : Inport  Port=4  SampleTime=t_sample
  user_gain : Inport  Port=5
  Bus Creator : BusCreator  Inputs=2
  Bus Selector : BusSelector  OutputSignals=NSIN_MIX,COS_MIX
  Bus Selector1 : BusSelector  OutputSignals=MAG_SET
  Data Type Conversion : DataTypeConversion  OutDataTypeStr=fixdt(1,16,15)  RndMeth=Nearest
  Data Type Conversion1 : DataTypeConversion  OutDataTypeStr=int16  ConvertRealWorld=Stored Integer (SI)  RndMeth=Nearest
  Data Type Conversion2 : DataTypeConversion  OutDataTypeStr=fixdt(1,18,16)  RndMeth=Nearest
  Data Type Conversion3 : DataTypeConversion  OutDataTypeStr=fixdt(1,18,16)  RndMeth=Nearest
  Product : Product  RndMeth=Nearest  SaturateOnIntegerOverflow=on
  Product1 : Product  RndMeth=Nearest  SaturateOnIntegerOverflow=on
  Product2 : Product  RndMeth=Nearest  SaturateOnIntegerOverflow=on
  Sum : Sum  OutDataTypeStr=fixdt(1,25,22)  RndMeth=Nearest  SaturateOnIntegerOverflow=on  SampleTime=t_sample  LockScale=on
  dac_o : Outport
  wires:
  Bus Selector/1 -> Product/2  "<NSIN_MIX>"
  Product/1 -> Sum/1
  Product1/1 -> Sum/2
  Bus Selector/2 -> Product1/1  "<COS_MIX>"
  mix_bus/1 -> Bus Selector/1  "phase_to_mux"
  Q/1 -> Data Type Conversion2/1
  Data Type Conversion/1 -> Data Type Conversion1/1
  valid/1 -> Bus Creator/2  "TVALID"
  Data Type Conversion1/1 -> Bus Creator/1  "TDATA"
  Bus Creator/1 -> dac_o/1
  Data Type Conversion3/1 -> Product1/2
  Data Type Conversion2/1 -> Product/1
  Sum/1 -> Product2/1
  Product2/1 -> Data Type Conversion/1
  I/1 -> Data Type Conversion3/1
  user_gain/1 -> Bus Selector1/1
  Bus Selector1/1 -> Product2/2  "<MAG_SET>"

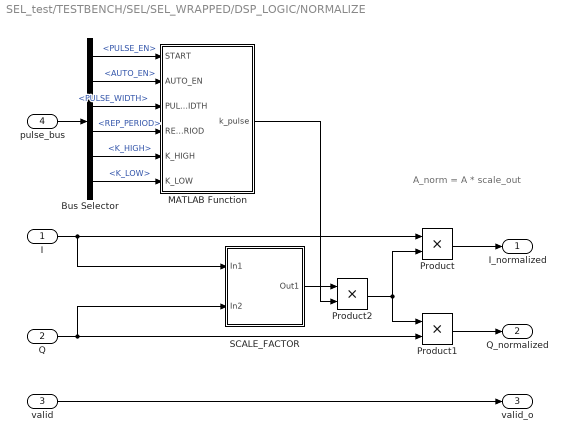
== system SEL_test/TESTBENCH/SEL/SEL_WRAPPED/DSP_LOGIC/NORMALIZE ==
  note: A_norm = A * scale_out
  I : Inport
  Q : Inport  Port=2
  valid : Inport  Port=3
  pulse_bus : Inport  Port=4
  Bus Selector : BusSelector  OutputSignals=PULSE_EN,AUTO_EN,PULSE_WIDTH,REP_PERIOD,K_HIGH,K_LOW
  MATLAB Function : MATLAB Function  TreatAsAtomicUnit=on
  Product : Product  OutDataTypeStr=fixdt(1,25,23)  RndMeth=Nearest  SaturateOnIntegerOverflow=on
  Product1 : Product  OutDataTypeStr=fixdt(1,25,23)  RndMeth=Nearest  SaturateOnIntegerOverflow=on
  Product2 : Product  OutDataTypeStr=fixdt(0,18,11)  RndMeth=Nearest  SaturateOnIntegerOverflow=on
  SCALE_FACTOR : Subsystem  TreatAsAtomicUnit=on
  I_normalized : Outport
  Q_normalized : Outport  Port=2
  valid_o : Outport  Port=3
  wires:
  I/1 -> Product/1, SCALE_FACTOR/1(In1)
  Q/1 -> Product1/2, SCALE_FACTOR/2(In2)
  Product/1 -> I_normalized/1
  Product1/1 -> Q_normalized/1
  valid/1 -> valid_o/1
  SCALE_FACTOR/1(Out1) -> Product2/1
  Product2/1 -> Product1/1, Product/2
  MATLAB Function/1(k_pulse) -> Product2/2
  pulse_bus/1 -> Bus Selector/1
  Bus Selector/5 -> MATLAB Function/5(K_HIGH)  "<K_HIGH>"
  Bus Selector/6 -> MATLAB Function/6(K_LOW)  "<K_LOW>"
  Bus Selector/3 -> MATLAB Function/3(PULSE_WIDTH)  "<PULSE_WIDTH>"
  Bus Selector/1 -> MATLAB Function/1(START)  "<PULSE_EN>"
  Bus Selector/2 -> MATLAB Function/2(AUTO_EN)  "<AUTO_EN>"
  Bus Selector/4 -> MATLAB Function/4(REP_PERIOD)  "<REP_PERIOD>"

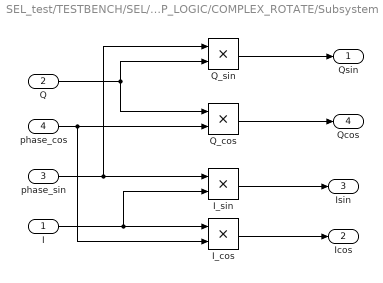
== system SEL_test/TESTBENCH/SEL/SEL_WRAPPED/DSP_LOGIC/COMPLEX_ROTATE/Subsystem ==
  I : Inport
  Q : Inport  Port=2
  phase_sin : Inport  Port=3
  phase_cos : Inport  Port=4
  I_cos : Product  OutDataTypeStr=fixdt(1,25,23)  RndMeth=Nearest  SaturateOnIntegerOverflow=on
  I_sin : Product  OutDataTypeStr=fixdt(1,25,23)  RndMeth=Nearest  SaturateOnIntegerOverflow=on
  Q_cos : Product  OutDataTypeStr=fixdt(1,25,23)  RndMeth=Nearest  SaturateOnIntegerOverflow=on
  Q_sin : Product  OutDataTypeStr=fixdt(1,25,23)  RndMeth=Nearest  SaturateOnIntegerOverflow=on
  Qsin : Outport
  Icos : Outport  Port=2
  Isin : Outport  Port=3
  Qcos : Outport  Port=4
  wires:
  I_cos/1 -> Icos/1
  Q/1 -> Q_sin/2, Q_cos/1
  phase_sin/1 -> Q_sin/1, I_sin/1
  I/1 -> I_sin/2, I_cos/1
  Q_sin/1 -> Qsin/1
  I_sin/1 -> Isin/1
  Q_cos/1 -> Qcos/1
  phase_cos/1 -> Q_cos/2, I_cos/2

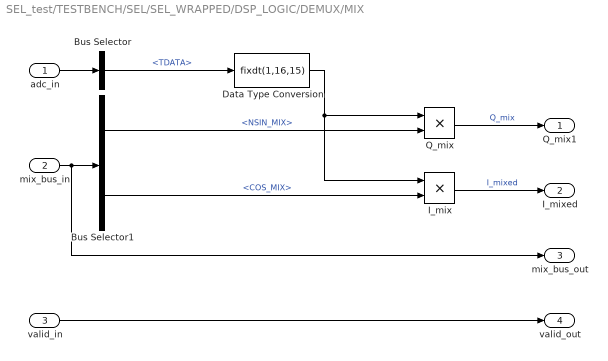
== system SEL_test/TESTBENCH/SEL/SEL_WRAPPED/DSP_LOGIC/DEMUX/MIX ==
  adc_in : Inport
  mix_bus_in : Inport  Port=2
  valid_in : Inport  Port=3
  Bus Selector : BusSelector  OutputSignals=TDATA
  Bus Selector1 : BusSelector  OutputSignals=NSIN_MIX,COS_MIX
  Data Type Conversion : DataTypeConversion  OutDataTypeStr=fixdt(1,16,15)  ConvertRealWorld=Stored Integer (SI)  RndMeth=Nearest
  I_mix : Product  OutDataTypeStr=fixdt(1,18,17)  RndMeth=Nearest  SaturateOnIntegerOverflow=on  LockScale=on
  Q_mix : Product  OutDataTypeStr=fixdt(1,18,17)  RndMeth=Nearest  SaturateOnIntegerOverflow=on  LockScale=on
  Q_mix1 : Outport
  I_mixed : Outport  Port=2
  mix_bus_out : Outport  Port=3  VectorParamsAs1DForOutWhenUnconnected=off
  valid_out : Outport  Port=4  VectorParamsAs1DForOutWhenUnconnected=off
  wires:
  Bus Selector1/1 -> Q_mix/2  "<NSIN_MIX>"
  Bus Selector1/2 -> I_mix/2  "<COS_MIX>"
  I_mix/1 -> I_mixed/1  "I_mixed"
  adc_in/1 -> Bus Selector/1
  mix_bus_in/1 -> mix_bus_out/1, Bus Selector1/1
  Q_mix/1 -> Q_mix1/1  "Q_mix"
  Bus Selector/1 -> Data Type Conversion/1  "<TDATA>"
  Data Type Conversion/1 -> Q_mix/1, I_mix/1
  valid_in/1 -> valid_out/1

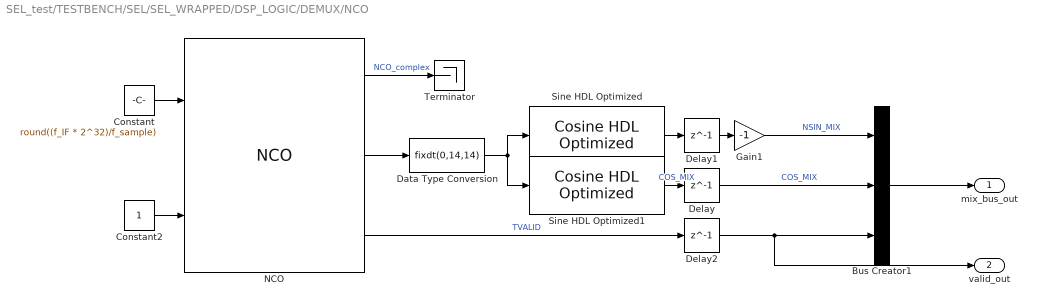
== system SEL_test/TESTBENCH/SEL/SEL_WRAPPED/DSP_LOGIC/DEMUX/NCO ==
  Bus Creator1 : BusCreator  Inputs=3
  Constant : Constant  Value=round((f_IF * 2^32)/f_sample)  OutDataTypeStr=fixdt(0,32,0)  SampleTime=t_sample
  Constant2 : Constant  OutDataTypeStr=boolean  SampleTime=-1
  Data Type Conversion : DataTypeConversion  OutDataTypeStr=fixdt(0,14,14)  ConvertRealWorld=Stored Integer (SI)  RndMeth=Nearest
  Delay : Delay  DelayLength=1  InitialCondition=0
  Delay1 : Delay  DelayLength=1  InitialCondition=0
  Delay2 : Delay  DelayLength=1  InitialCondition=0
  Gain1 : Gain  Gain=-1  RndMeth=Nearest  SaturateOnIntegerOverflow=on  OutDataTypeStr=Inherit: Same as input
  NCO : dsphdlsigops2/NCO  PhaseIncrementSource=Input port  PhaseIncrement=round((f_IF/f_sample) * 2^24)  Frequency=510  FreqResolution=0.05  SamplingFreq=4000  PhaseOffsetSource=Property  PhaseOffset=0  PhaseOffsetR=pi/3  DitherSource=Property  NumDitherBits=4  SamplesPerFrame=1  LUTCompress=off  ResetAction=off  Waveform=Sine  PhasePort=on  SimulateUsing=Code generation  AccumulatorWL=32  PhaseQuantization=on  NumQuantizerAccumulatorBits=14  OutputDataType=Binary point scaling  OutputWL=16  OutputFL=15
  Sine HDL Optimized : hdlsllib/Lookup Tables/Cosine HDL Optimized  OutputFormula=sin(2*pi*u)  NumDataPoints=2^(14-2)  TableDataTypeStr=fixdt(0,24,23)  SimulateLUTROMDelay=off
      settings: LibrarySourceBlock=|
      | hdlsllib/Lookup
      | Tables/Sine
      | HDL Optimized
  Sine HDL Optimized1 : hdlsllib/Lookup Tables/Cosine HDL Optimized  OutputFormula=cos(2*pi*u)  NumDataPoints=2^(14-2)  TableDataTypeStr=fixdt(0,24,23)  SimulateLUTROMDelay=off
      settings: LibrarySourceBlock=|
      | hdlsllib/Lookup
      | Tables/Sine
      | HDL Optimized
  Terminator : Terminator
  mix_bus_out : Outport  VectorParamsAs1DForOutWhenUnconnected=off
  valid_out : Outport  Port=2  VectorParamsAs1DForOutWhenUnconnected=off
  wires:
  Constant2/1 -> NCO/2
  NCO/3 -> Delay2/1  "TVALID"
  Constant/1 -> NCO/1
  NCO/1 -> Terminator/1  "NCO_complex"
  Data Type Conversion/1 -> Sine HDL Optimized1/1, Sine HDL Optimized/1
  Gain1/1 -> Bus Creator1/1  "NSIN_MIX"
  Sine HDL Optimized1/1 -> Delay/1  "COS_MIX"
  Bus Creator1/1 -> mix_bus_out/1
  NCO/2 -> Data Type Conversion/1
  Sine HDL Optimized/1 -> Delay1/1
  Delay1/1 -> Gain1/1
  Delay/1 -> Bus Creator1/2  "COS_MIX"
  Delay2/1 -> Bus Creator1/3, valid_out/1

== system SEL_test/TESTBENCH/SEL/SEL_WRAPPED/DSP_LOGIC/NORMALIZE/SCALE_FACTOR ==
  note: S_in = I^2 + Q^2
  In1 : Inport
  In2 : Inport  Port=2
  Data Type Conversion1 : DataTypeConversion  OutDataTypeStr=fixdt(1,18,16)  RndMeth=Nearest
  Data Type Conversion2 : DataTypeConversion  OutDataTypeStr=fixdt(1,18,16)  RndMeth=Nearest
  Product : Product  RndMeth=Nearest  SaturateOnIntegerOverflow=on
  Product1 : Product  RndMeth=Nearest  SaturateOnIntegerOverflow=on
  Sum : Sum  RndMeth=Nearest  SaturateOnIntegerOverflow=on
  rSqrt : Subsystem
  Out1 : Outport
  wires:
  Product1/1 -> Sum/2
  In1/1 -> Data Type Conversion2/1
  rSqrt/1(K) -> Out1/1  "rsqrt"
  In2/1 -> Data Type Conversion1/1
  Product/1 -> Sum/1
  Data Type Conversion2/1 -> Product/1, Product/2
  Data Type Conversion1/1 -> Product1/2, Product1/1
  Sum/1 -> rSqrt/1(S_in)

== system SEL_test/TESTBENCH/SEL/SEL_WRAPPED/DSP_LOGIC/NORMALIZE/SCALE_FACTOR/rSqrt ==
  note: Post Shift:
      | lut_output << m
      | cast to uint18_en10
  note: rSqrt LUT:
      | parity = 0, return 1/sqrt(address)
      | parity = 1, return sqrt(2)/sqrt(address)
  note: Leading Zero Count:
      | LZC = k
      | x_norm = x_in << k
      | m = k>>1
      | r = k & 1
      | addr = [r, 11address bits]
  S_in : Inport
  Data Type Conversion : DataTypeConversion  OutDataTypeStr=fixdt(0,28,27)  RndMeth=Nearest
  MATLAB Function : MATLAB Function  TreatAsAtomicUnit=on
  MATLAB Function1 : MATLAB Function  TreatAsAtomicUnit=on
  MOVING_AVG : Subsystem
  NORMALIZED_LUT : Lookup_n-D  NumberOfTableDimensions=1  LookupTableObject=''  BreakpointsForDimension1=uint16(0:2^12-1)  BreakpointsForDimension1FirstPoint=10  BreakpointsForDimension2FirstPoint=10  BreakpointsForDimension1Spacing=12  BreakpointsForDimension2Spacing=12  BreakpointsForDimension1DataTypeStr=Inherit: Inherit from 'Breakpoint data'  IndexSearchMethod=Evenly spaced points  Table=lut_rSqrt  TableDataTypeStr=Inherit: Inherit from 'Table data'  InterpMethod=Flat  DiagnosticForOutOfRangeInput=Error  RemoveProtectionInput=on  InternalRulePriority=Speed  OutDataTypeStr=Inherit: Inherit from 'Table data'  RndMeth=Simplest
  K : Outport
  wires:
  Data Type Conversion/1 -> MOVING_AVG/1(In1)  "Converted_test_in"
  MOVING_AVG/1(S_in) -> MATLAB Function/1(x_in)  "Smoothed_test_in"
  MATLAB Function/1(lut_addr_12bit) -> NORMALIZED_LUT/1  "lut_addr_12bit"
  NORMALIZED_LUT/1 -> MATLAB Function1/1(lut_val_16bit)  "lut_output"
  MATLAB Function/2(m) -> MATLAB Function1/2(m)  "m"
  MATLAB Function1/1(K) -> K/1  "final_scale_factor"
  S_in/1 -> Data Type Conversion/1

== system SEL_test/TESTBENCH/SEL/SEL_WRAPPED/DSP_LOGIC/NORMALIZE/SCALE_FACTOR/rSqrt/MOVING_AVG ==
  In1 : Inport
  Gain : Gain  Gain=1/2  OutDataTypeStr=fixdt(0,28,27)  RndMeth=Nearest  SaturateOnIntegerOverflow=on
  Sum : Sum  Inputs=|++  RndMeth=Nearest  SaturateOnIntegerOverflow=on
  Unit Delay : UnitDelay  SampleTime=-1
  S_in : Outport
  wires:
  Sum/1 -> Gain/1
  In1/1 -> Sum/2, Unit Delay/1
  Unit Delay/1 -> Sum/1
  Gain/1 -> S_in/1

== matlab function SEL_test/TESTBENCH/SEL/SEL_WRAPPED/DSP_LOGIC/NORMALIZE/SCALE_FACTOR/rSqrt/MATLAB Function ==
  data: x_in input; lut_addr_12bit output; m output
function [lut_addr_12bit, m] = lzc_and_normalize(x_in)
%#codegen
% x_in is ufix28_en27 (28 bits total, 27 fractional bits)
%   Bit 28: 2^0 = 1.0 (Full Scale Power)
%   Bits 27..1: 2^-1 down to 2^-27

% 1. Extract raw 28-bit integer into a 32-bit container
x_int = uint32(storedInteger(x_in));

% 2. Priority Encoder for Leading Zero Count (LZC)
% k measures shift count to align the leading '1' to Bit 28 (2^0)
if bitget(x_int, 28) == 1
    k = uint16(0);
elseif bitget(x_int, 27) == 1
    k = uint16(1);
elseif bitget(x_int, 26) == 1
    k = uint16(2);
elseif bitget(x_int, 25) == 1
    k = uint16(3);
elseif bitget(x_int, 24) == 1
    k = uint16(4);
elseif bitget(x_int, 23) == 1
    k = uint16(5);
elseif bitget(x_int, 22) == 1
    k = uint16(6);
elseif bitget(x_int, 21) == 1
    k = uint16(7);
elseif bitget(x_int, 20) == 1
    k = uint16(8);
elseif bitget(x_int, 19) == 1
    k = uint16(9);
elseif bitget(x_int, 18) == 1
    k = uint16(10);
elseif bitget(x_int, 17) == 1
    k = uint16(11);
elseif bitget(x_int, 16) == 1
    k = uint16(12);
elseif bitget(x_int, 15) == 1
    k = uint16(13);
elseif bitget(x_int, 14) == 1
    k = uint16(14);
elseif bitget(x_int, 13) == 1
    k = uint16(15);
elseif bitget(x_int, 12) == 1
    k = uint16(16);
elseif bitget(x_int, 11) == 1
    k = uint16(17);
elseif bitget(x_int, 10) == 1
    k = uint16(18);
elseif bitget(x_int, 9) == 1
    k = uint16(19);
elseif bitget(x_int, 8) == 1
    k = uint16(20);
elseif bitget(x_int, 7) == 1
    k = uint16(21);
elseif bitget(x_int, 6) == 1
    k = uint16(22);
elseif bitget(x_int, 5) == 1
    k = uint16(23);
elseif bitget(x_int, 4) == 1
    k = uint16(24);
elseif bitget(x_int, 3) == 1
    k = uint16(25);
elseif bitget(x_int, 2) == 1
    k = uint16(26);
elseif bitget(x_int, 1) == 1
    k = uint16(27);
else
    k = uint16(27); % Zero clamp
end

% 3. Extract post-LUT shift m and parity bit r
m = bitshift(k, -1);                  % k >> 1 (m ranges from 0 to 13)
r = bitand(k, uint16(1));             % k & 1

% 4. Normalize input: shift left so leading '1' lands on Bit 28
x_norm = bitshift(x_int, k);

% 5. Extract top 11 fractional bits (Bits 27 down to 17)
% Shift right by 16 moves Bit 17 to Bit 1, mask with 2047 (0x07FF)
frac_11bit = bitand(uint16(bitshift(x_norm, -16)), uint16(2047));

% 6. Combine parity bit r (Bit 12) with 11-bit address (Bits 11..1)
lut_addr_12bit = bitor(bitshift(r, 11), frac_11bit);
end

== matlab function SEL_test/TESTBENCH/SEL/SEL_WRAPPED/DSP_LOGIC/NORMALIZE/MATLAB Function ==
  settings: fimath=fimath('RoundingMethod', 'Floor','OverflowAction', 'Wrap','ProductMode', 'FullPrecision', 'SumMode', 'FullPrecision')
  data: START input; k_pulse output; AUTO_EN input; PULSE_WIDTH input; REP_PERIOD input; K_HIGH input; K_LOW input
function k_pulse = KPulseGenerator(START, AUTO_EN, PULSE_WIDTH, REP_PERIOD, K_HIGH, K_LOW)
%#codegen
%
% Configurable Hardware Pulse Generator for SEL Loop Control
% Outputs k_pulse to scale normalized I/Q vectors without breaking phase lock.
%
% Inputs:
%   START       : Single-shot trigger (PULSE_EN) from AXI register (Boolean)
%   AUTO_EN     : Continuous repeating mode toggle (Boolean)
%   PULSE_WIDTH : Pulse ON duration in clock cycles (uint32)
%   REP_PERIOD  : Total period (ON + OFF) in clock cycles (uint32)
%   K_HIGH      : Pulse ON scale factor, typical 1.0 (sfix18_En16)
%   K_LOW       : Pulse OFF scale factor, e.g., 0.0 or 0.01 keep-alive (sfix18_En16)
%
% Output:
%   k_pulse     : Pulsed multiplier value (sfix18_En16)

persistent pulse_active start_prev pulse_count rep_count
if isempty(pulse_active)
    pulse_active = false;
    start_prev   = false;
    pulse_count  = uint32(0);
    rep_count    = uint32(0);
end

% -------------------------------------------------------------------------
% 1. Trigger Detection
% -------------------------------------------------------------------------
% Single-shot rising edge trigger
start_pulse = START && ~start_prev;
start_prev  = START;

% Continuous repetition auto-trigger
auto_trigger = false;
if AUTO_EN && (REP_PERIOD > uint32(0))
    if rep_count >= (REP_PERIOD - uint32(1))
        rep_count    = uint32(0);
        auto_trigger = true;
    else
        rep_count = rep_count + uint32(1);
    end
else
    rep_count = uint32(0);
end

% Combined trigger condition
if start_pulse || auto_trigger
    pulse_active = true;
    pulse_count  = uint32(0);
end

% -------------------------------------------------------------------------
% 2. Pulse Output State Machine
% -------------------------------------------------------------------------
if pulse_active
    if pulse_count < PULSE_WIDTH
        % Active ON state
        k_pulse     = K_HIGH;
        pulse_count = pulse_count + uint32(1);
    else
        % Pulse width elapsed -> transition to OFF
        k_pulse      = K_LOW;
        pulse_active = false;
        pulse_count  = uint32(0);
    end
else
    % Idle / OFF state
    k_pulse = K_LOW;
end

end

== matlab function SEL_test/TESTBENCH/SEL/SEL_WRAPPED/DSP_LOGIC/NORMALIZE/SCALE_FACTOR/rSqrt/MATLAB Function1 ==
  data: lut_val_16bit input; K output; m input
function K = apply_post_shift(lut_val_16bit, m)
%#codegen
% lut_val_16bit : ufix16_en15 (16 bits from LUT)
% m              : uint16 [0..13]
% K              : ufix18_en4 (18-bit Word Length for DSP slice, max gain 16383.9)

% 1. Extract raw 16-bit integer into 32-bit container to prevent shift overflow
N_lut = uint32(storedInteger(lut_val_16bit));

% 2. Dynamic left shift by m (m ranges from 0 to 13)
N_shifted = bitshift(N_lut, uint32(m));

% 3. Truncate 11 LSBs to transition from en15 -> en4 (15 - 4 = 11)
N_final = bitshift(N_shifted, -11); 

% 4. Store in 18-bit container & re-interpret bit pattern as ufix18_en4
raw18 = fi(N_final, 0, 18, 0);
T_out = numerictype(0, 18, 4);

K = reinterpretcast(raw18, T_out);
end
